simulink model "lab3_postlab2"  (R2016a)
settings: Solver=VariableStepAuto  StartTime=0.0  StopTime=500  RelTol=1e-3
values from neighbouring files (symbols this model uses):
  C_D = H'    [lab3_sumup.m]
  G_D = G'    [lab3_sumup.m]
  Gcl = dcgain(sys5)    [lab3_sumup.m]
  H_D = C'    [lab3_sumup.m]
  K = K'    [lab3_sumup.m]
  L_ndb = acker(G_D, H_D, [p0, p1])    [lab3_sumup.m]
  Ts = 0.75    [lab3_sumup.m]
  x = [0 0.3]'    [lab3_sumup.m]
libraries: simulink x1
settings Model: Creator=Helvins  LastModifiedBy=Helvins

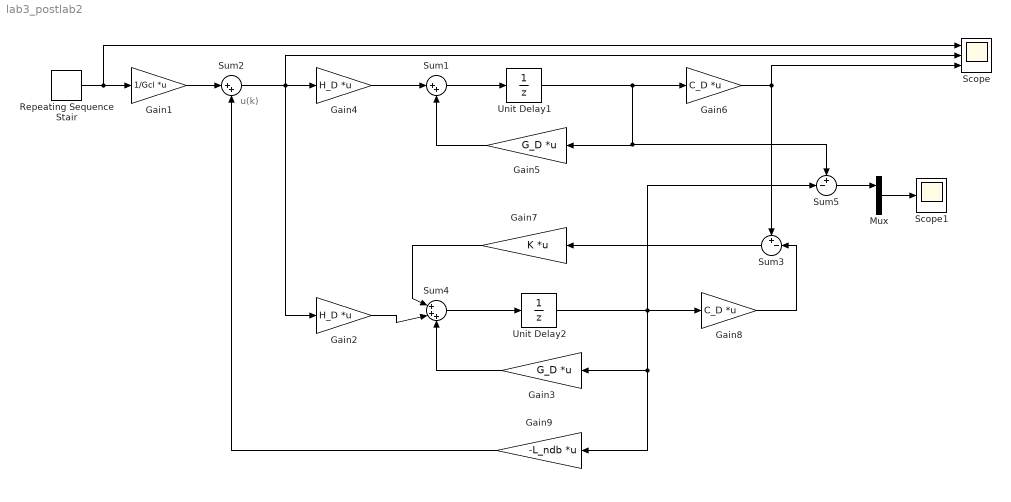
== system lab3_postlab2 ==
  note: u(k)
  Gain1 : Gain  Gain=1/Gcl  Multiplication=Matrix(K*u)
  Gain2 : Gain  Gain=H_D  Multiplication=Matrix(K*u)
  Gain3 : Gain  Gain=G_D  Multiplication=Matrix(K*u)
  Gain4 : Gain  Gain=H_D  Multiplication=Matrix(K*u)
  Gain5 : Gain  Gain=G_D  Multiplication=Matrix(K*u)
  Gain6 : Gain  Gain=C_D  Multiplication=Matrix(K*u)
  Gain7 : Gain  Gain=K  Multiplication=Matrix(K*u)
  Gain8 : Gain  Gain=C_D  Multiplication=Matrix(K*u)
  Gain9 : Gain  Gain=-L_ndb  Multiplication=Matrix(K*u)
  Mux : Mux  Inputs=2
  Repeating Sequence Stair : simulink/Sources/Repeating Sequence Stair  OutValues=[0, 0.7, -0.2, 0.5, 0].'  tsamp=140*Ts  OutMin=[]  OutMax=[]  OutDataTypeStr=double  OutputDataTypeScalingMode=double  OutDataType=fixdt(0,8)  ConRadixGroup=Best Precision: Vector-wise  OutScaling=2^-12
  Scope : Scope  NumInputPorts=3
  Scope1 : Scope
  Sum1 : Sum  Inputs=|++
  Sum2 : Sum  Inputs=|++
  Sum3 : Sum  Inputs=+-|
  Sum4 : Sum  Inputs=|+++
  Sum5 : Sum  Inputs=+-|
  Unit Delay1 : UnitDelay  InitialCondition=[x(1); x(2)]  SampleTime=Ts
  Unit Delay2 : UnitDelay  InitialCondition=[0; 0]  SampleTime=Ts
  wires:
  Gain4/1 -> Sum1/1
  Gain5/1 -> Sum1/2
  Sum1/1 -> Unit Delay1/1
  Unit Delay1/1 -> Sum5/1, Gain5/1, Gain6/1
  Sum2/1 -> Gain2/1, Scope/2, Gain4/1
  Gain1/1 -> Sum2/1
  Repeating Sequence Stair/1 -> Scope/1, Gain1/1
  Gain6/1 -> Scope/3, Sum3/1
  Unit Delay2/1 -> Sum5/2, Gain9/1, Gain3/1, Gain8/1
  Gain8/1 -> Sum3/2
  Sum3/1 -> Gain7/1
  Gain7/1 -> Sum4/1
  Gain2/1 -> Sum4/2
  Gain3/1 -> Sum4/3
  Sum4/1 -> Unit Delay2/1
  Gain9/1 -> Sum2/2
  Mux/1 -> Scope1/1
  Sum5/1 -> Mux/1
